simulink model "w31_v6"  (Simulink 7.9)
settings: Solver=FixedStepDiscrete  StartTime=0.0  StopTime=inf  FixedStep=0.01  RelTol=1e-3
undefined symbols (not defined in the file): DiscIntNeverNeededParam, magnitude
libraries: canmsglib x24, cansrvlib x22, simulink x12, iohwablib x5, legionoslib x3, ccpsrvlib x2, memsrvlib x1, tgttoollib x1, udssrvlib x1, wdgmlib x1
(part 5 of 5)

== stateflow chart CAN_Receive_10ms/Remote_Control_CAN/Remote_IO_situation1/Chart ==
  state MsgNotRecieve
    en:
    NoRxMsgComfirm=0;
    du:
    NoRxMsgCnt++;
  state MsgRecieve
    en:
    NoRxMsgCnt=0;
    NoRxMsgComfirm=0;
  state MsgNotRecieveComfirm
    en:
    NoRxMsgComfirm=1;
    du:
    NoRxMsgCnt++;
  note: NoRxMsgCnt在RxMsg==0的情况下（CAN信息没有在规定的周期内及时更新）
      | 一直往上加，直到RxMsg==1，NoRxMsgCnt清零。（程序接收到新的CAN信息）。NoRxMsgCnt只受到RxMsg控制。
  note: NoRxMsgComfirm受NoRxMsgCnt和NoRxMsgCntMax两个量控制
      | NoRxmsgComfirm==1没有接收到消息
  state NoRxMsgCntOverFlow
    en:
    NoRxMsgCnt=65000;
  (default) -> MsgNotRecieve : {NoRxMsgCnt=0;}
  MsgNotRecieve -> MsgRecieve [order 1] : [1==RxMsg]
  NoRxMsgCntOverFlow -> MsgRecieve : [1==RxMsg]
  MsgRecieve -> MsgNotRecieve : [0==RxMsg]
  MsgNotRecieveComfirm -> MsgRecieve [order 1] : [1==RxMsg]
  MsgNotRecieve -> MsgNotRecieveComfirm [order 2] : [NoRxMsgCnt>NoRxMsgCntMax]
  MsgNotRecieveComfirm -> NoRxMsgCntOverFlow [order 2] : [NoRxMsgCnt>=65000]
  data: NoRxMsgComfirm output boolean; RxMsg input boolean; NoRxMsgCnt output single; NoRxMsgCntMax input single

== stateflow chart CAN_Receive_10ms/Chassis_CAN/RL_Motor_NoMsg/Chart ==
  state MsgNotRecieve
    en:
    NoRxMsgComfirm=0;
    du:
    NoRxMsgCnt++;
  state MsgRecieve
    en:
    NoRxMsgCnt=0;
    NoRxMsgComfirm=0;
  state MsgNotRecieveComfirm
    en:
    NoRxMsgComfirm=1;
    du:
    NoRxMsgCnt++;
  note: NoRxMsgCnt在RxMsg==0的情况下（CAN信息没有在规定的周期内及时更新）
      | 一直往上加，直到RxMsg==1，NoRxMsgCnt清零。（程序接收到新的CAN信息）。NoRxMsgCnt只受到RxMsg控制。
  note: NoRxMsgComfirm受NoRxMsgCnt和NoRxMsgCntMax两个量控制
      | NoRxmsgComfirm==1没有接收到消息
  state NoRxMsgCntOverFlow
    en:
    NoRxMsgCnt=65000;
  (default) -> MsgNotRecieve : {NoRxMsgCnt=0;}
  MsgNotRecieve -> MsgRecieve [order 1] : [1==RxMsg]
  NoRxMsgCntOverFlow -> MsgRecieve : [1==RxMsg]
  MsgRecieve -> MsgNotRecieve : [0==RxMsg]
  MsgNotRecieveComfirm -> MsgRecieve [order 1] : [1==RxMsg]
  MsgNotRecieve -> MsgNotRecieveComfirm [order 2] : [NoRxMsgCnt>NoRxMsgCntMax]
  MsgNotRecieveComfirm -> NoRxMsgCntOverFlow [order 2] : [NoRxMsgCnt>=65000]
  data: NoRxMsgComfirm output boolean; RxMsg input boolean; NoRxMsgCnt output single; NoRxMsgCntMax input single

== stateflow chart CAN_Receive_10ms/Chassis_CAN/RR_Motor_NoMsg/Chart ==
  state MsgNotRecieve
    en:
    NoRxMsgComfirm=0;
    du:
    NoRxMsgCnt++;
  state MsgRecieve
    en:
    NoRxMsgCnt=0;
    NoRxMsgComfirm=0;
  state MsgNotRecieveComfirm
    en:
    NoRxMsgComfirm=1;
    du:
    NoRxMsgCnt++;
  note: NoRxMsgCnt在RxMsg==0的情况下（CAN信息没有在规定的周期内及时更新）
      | 一直往上加，直到RxMsg==1，NoRxMsgCnt清零。（程序接收到新的CAN信息）。NoRxMsgCnt只受到RxMsg控制。
  note: NoRxMsgComfirm受NoRxMsgCnt和NoRxMsgCntMax两个量控制
      | NoRxmsgComfirm==1没有接收到消息
  state NoRxMsgCntOverFlow
    en:
    NoRxMsgCnt=65000;
  (default) -> MsgNotRecieve : {NoRxMsgCnt=0;}
  MsgNotRecieve -> MsgRecieve [order 1] : [1==RxMsg]
  NoRxMsgCntOverFlow -> MsgRecieve : [1==RxMsg]
  MsgRecieve -> MsgNotRecieve : [0==RxMsg]
  MsgNotRecieveComfirm -> MsgRecieve [order 1] : [1==RxMsg]
  MsgNotRecieve -> MsgNotRecieveComfirm [order 2] : [NoRxMsgCnt>NoRxMsgCntMax]
  MsgNotRecieveComfirm -> NoRxMsgCntOverFlow [order 2] : [NoRxMsgCnt>=65000]
  data: NoRxMsgComfirm output boolean; RxMsg input boolean; NoRxMsgCnt output single; NoRxMsgCntMax input single

== matlab function Logic_And_Algorithm/Remote_mode_with_control_2/Power_calculation/Speed distribution strategy/speed gear slection ==
  data: u1 input double; y output double; u2 input double
function y = fcn(u1,u2)
%#codegen
%这个程序是用来做挡位控制的，目前希望是一档0-5，二档0-20，三档0-40.
if (u1==0)
    y = (5/30)*u2;

elseif(u1 == 1)
        y = (10/30)*u2;
        
else 
        y = (20/30)*u2;

end

y=u2;

end

== matlab function Logic_And_Algorithm/Remote_mode_with_control_0/Power_calculation/Speed distribution strategy/motion distribution1/Switch Case Action Subsystem/MATLAB Function ==
  data: steering_wheel_angle_dem input double; gain1 output double; gain2 output double; gain3 output double; gain4 output double
function [gain1,gain2,gain3,gain4] = fcn(steering_wheel_angle_dem)
%#codegen
%现进行逻辑说明，规定左转为正，右转为负，当前轮减后轮为正的时候，车辆左转，此时gain为逆时针原地转向；
%差值为负时，车辆右转，此时gain为顺时针原地转向

initial_gain=1;
gain1=initial_gain;
gain2=initial_gain;
gain3=initial_gain;
gain4=initial_gain;

if (steering_wheel_angle_dem>=0)
    gain1=-1;gain3=-1;
    gain2=1;gain4=1;
else
    gain1=1;gain3=1;
    gain2=-1;gain4=-1;
end

end

== stateflow chart CAN_Receive_10ms/iECU_CAN/shake_situation1/Chart ==
  state MsgNotRecieve
    en:
    NoRxMsgComfirm=0;
    du:
    NoRxMsgCnt++;
  state MsgRecieve
    en:
    NoRxMsgCnt=0;
    NoRxMsgComfirm=0;
  state MsgNotRecieveComfirm
    en:
    NoRxMsgComfirm=1;
    du:
    NoRxMsgCnt++;
  note: NoRxMsgCnt在RxMsg==0的情况下（CAN信息没有在规定的周期内及时更新）
      | 一直往上加，直到RxMsg==1，NoRxMsgCnt清零。（程序接收到新的CAN信息）。NoRxMsgCnt只受到RxMsg控制。
  note: NoRxMsgComfirm受NoRxMsgCnt和NoRxMsgCntMax两个量控制
      | NoRxmsgComfirm==1没有接收到消息
  state NoRxMsgCntOverFlow
    en:
    NoRxMsgCnt=65000;
  (default) -> MsgNotRecieve : {NoRxMsgCnt=0;}
  MsgNotRecieve -> MsgRecieve [order 1] : [1==RxMsg]
  NoRxMsgCntOverFlow -> MsgRecieve : [1==RxMsg]
  MsgRecieve -> MsgNotRecieve : [0==RxMsg]
  MsgNotRecieveComfirm -> MsgRecieve [order 1] : [1==RxMsg]
  MsgNotRecieve -> MsgNotRecieveComfirm [order 2] : [NoRxMsgCnt>NoRxMsgCntMax]
  MsgNotRecieveComfirm -> NoRxMsgCntOverFlow [order 2] : [NoRxMsgCnt>=65000]
  data: NoRxMsgComfirm output boolean; RxMsg input boolean; NoRxMsgCnt output single; NoRxMsgCntMax input single

== matlab function Logic_And_Algorithm/iECU_mode_with_control/Power_calculation/Speed distribution strategy/MATLAB Function ==
  data: u1 input double; y output double; u2 input double
function y = fcn(u1,u2)
%#codegen

if (u1 == 2 && u2 <= 20)
        y = u2;

elseif(u1 == 2 && u2 > 20)
        y = 20;        
        
elseif (u1==1 && u2 <= 10)
       y = u2;

elseif(u1 == 1 && u2 > 10)
        y = 10;    
        
elseif (u1==0 && u2 <= 5)
      y = u2;

else
       y = 5;            

end

== matlab function Logic_And_Algorithm/Remote_mode_with_control_0/Power_calculation/Speed distribution strategy/MATLAB Function ==
  data: delta_f input double; nan_code output double; delta_r input double; mode input double
function nan_code = fcn(delta_f,delta_r,mode)
%#codegen
%进行逻辑说明，如果判断在运算过程中会出现NAN的情况，则在此处将nan_code的值置为1，选择均分动力输出，
%否则nan_code=0，选择计算结果输出

initial_code=0;
nan_code=initial_code;

if (mode==0)&&(delta_f==delta_r)
    nan_code=1;
else if (mode==3)&&(delta_f==0)&&(delta_r==0)
        nan_code=1;
    else if (mode==2)&&(delta_r==0)
            nan_code=1;
        else if (mode==1)&&(delta_f==0)
                nan_code=1;
            else if (mode==4)
                    nan_code=0;
                
                end
            end
        end
    end
end

end

== stateflow chart CAN_Receive_10ms/BMS_CAN/shake_situation1/Chart ==
  state MsgNotRecieve
    en:
    NoRxMsgComfirm=0;
    du:
    NoRxMsgCnt++;
  state MsgRecieve
    en:
    NoRxMsgCnt=0;
    NoRxMsgComfirm=0;
  state MsgNotRecieveComfirm
    en:
    NoRxMsgComfirm=1;
    du:
    NoRxMsgCnt++;
  note: NoRxMsgCnt在RxMsg==0的情况下（CAN信息没有在规定的周期内及时更新）
      | 一直往上加，直到RxMsg==1，NoRxMsgCnt清零。（程序接收到新的CAN信息）。NoRxMsgCnt只受到RxMsg控制。
  note: NoRxMsgComfirm受NoRxMsgCnt和NoRxMsgCntMax两个量控制
      | NoRxmsgComfirm==1没有接收到消息
  state NoRxMsgCntOverFlow
    en:
    NoRxMsgCnt=65000;
  (default) -> MsgNotRecieve : {NoRxMsgCnt=0;}
  MsgNotRecieve -> MsgRecieve [order 1] : [1==RxMsg]
  NoRxMsgCntOverFlow -> MsgRecieve : [1==RxMsg]
  MsgRecieve -> MsgNotRecieve : [0==RxMsg]
  MsgNotRecieveComfirm -> MsgRecieve [order 1] : [1==RxMsg]
  MsgNotRecieve -> MsgNotRecieveComfirm [order 2] : [NoRxMsgCnt>NoRxMsgCntMax]
  MsgNotRecieveComfirm -> NoRxMsgCntOverFlow [order 2] : [NoRxMsgCnt>=65000]
  data: NoRxMsgComfirm output boolean; RxMsg input boolean; NoRxMsgCnt output single; NoRxMsgCntMax input single

== matlab function Logic_And_Algorithm/Remote_mode_with_control_0/Power_calculation/Speed distribution strategy/motion distribution1/front steering/MATLAB Function ==
  data: fl input double; motion_fl output double; fr input double; rl input double; rr input double; motion_dem input double; motion_fr output double; motion_rl output double; motion_rr output double
function [motion_fl,motion_fr,motion_rl,motion_rr] = fcn(fl,fr,rl,rr,motion_dem)
%#codegen
%逻辑说明，四轮的实际请求速度应该乘以4，所以此处有一个对应的语句，
%目前由于在前后轮转角输入都为0的情况下无法正常计算，输出会为NaN，因此在此进行判断，若有NaN的输出则均分动力

if isnan(fl)||isnan(fr)||isnan(rl)||isnan(rr)
    motion_fl=motion_dem;
    motion_fr=motion_dem;
    motion_rl=motion_dem;
    motion_rr=motion_dem;
else
    motion_fl=fl*4;
    motion_fr=fr*4;
    motion_rl=rl*4;
    motion_rr=rr*4;
end
end

== stateflow chart CAN_Receive_10ms/Chassis_CAN/DBSF_NoMsg/Chart ==
  state MsgNotRecieve
    en:
    NoRxMsgComfirm=0;
    du:
    NoRxMsgCnt++;
  state MsgRecieve
    en:
    NoRxMsgCnt=0;
    NoRxMsgComfirm=0;
  state MsgNotRecieveComfirm
    en:
    NoRxMsgComfirm=1;
    du:
    NoRxMsgCnt++;
  note: NoRxMsgCnt在RxMsg==0的情况下（CAN信息没有在规定的周期内及时更新）
      | 一直往上加，直到RxMsg==1，NoRxMsgCnt清零。（程序接收到新的CAN信息）。NoRxMsgCnt只受到RxMsg控制。
  note: NoRxMsgComfirm受NoRxMsgCnt和NoRxMsgCntMax两个量控制
      | NoRxmsgComfirm==1没有接收到消息
  state NoRxMsgCntOverFlow
    en:
    NoRxMsgCnt=65000;
  (default) -> MsgNotRecieve : {NoRxMsgCnt=0;}
  MsgNotRecieve -> MsgRecieve [order 1] : [1==RxMsg]
  NoRxMsgCntOverFlow -> MsgRecieve : [1==RxMsg]
  MsgRecieve -> MsgNotRecieve : [0==RxMsg]
  MsgNotRecieveComfirm -> MsgRecieve [order 1] : [1==RxMsg]
  MsgNotRecieve -> MsgNotRecieveComfirm [order 2] : [NoRxMsgCnt>NoRxMsgCntMax]
  MsgNotRecieveComfirm -> NoRxMsgCntOverFlow [order 2] : [NoRxMsgCnt>=65000]
  data: NoRxMsgComfirm output boolean; RxMsg input boolean; NoRxMsgCnt output single; NoRxMsgCntMax input single

== stateflow chart CAN_Receive_10ms/Chassis_CAN/EPSF_NoMsg/Chart ==
  state MsgNotRecieve
    en:
    NoRxMsgComfirm=0;
    du:
    NoRxMsgCnt++;
  state MsgRecieve
    en:
    NoRxMsgCnt=0;
    NoRxMsgComfirm=0;
  state MsgNotRecieveComfirm
    en:
    NoRxMsgComfirm=1;
    du:
    NoRxMsgCnt++;
  note: NoRxMsgCnt在RxMsg==0的情况下（CAN信息没有在规定的周期内及时更新）
      | 一直往上加，直到RxMsg==1，NoRxMsgCnt清零。（程序接收到新的CAN信息）。NoRxMsgCnt只受到RxMsg控制。
  note: NoRxMsgComfirm受NoRxMsgCnt和NoRxMsgCntMax两个量控制
      | NoRxmsgComfirm==1没有接收到消息
  state NoRxMsgCntOverFlow
    en:
    NoRxMsgCnt=65000;
  (default) -> MsgNotRecieve : {NoRxMsgCnt=0;}
  MsgNotRecieve -> MsgRecieve [order 1] : [1==RxMsg]
  NoRxMsgCntOverFlow -> MsgRecieve : [1==RxMsg]
  MsgRecieve -> MsgNotRecieve : [0==RxMsg]
  MsgNotRecieveComfirm -> MsgRecieve [order 1] : [1==RxMsg]
  MsgNotRecieve -> MsgNotRecieveComfirm [order 2] : [NoRxMsgCnt>NoRxMsgCntMax]
  MsgNotRecieveComfirm -> NoRxMsgCntOverFlow [order 2] : [NoRxMsgCnt>=65000]
  data: NoRxMsgComfirm output boolean; RxMsg input boolean; NoRxMsgCnt output single; NoRxMsgCntMax input single

== stateflow chart CAN_Receive_10ms/Chassis_CAN/EPSR_NoMsg/Chart ==
  state MsgNotRecieve
    en:
    NoRxMsgComfirm=0;
    du:
    NoRxMsgCnt++;
  state MsgRecieve
    en:
    NoRxMsgCnt=0;
    NoRxMsgComfirm=0;
  state MsgNotRecieveComfirm
    en:
    NoRxMsgComfirm=1;
    du:
    NoRxMsgCnt++;
  note: NoRxMsgCnt在RxMsg==0的情况下（CAN信息没有在规定的周期内及时更新）
      | 一直往上加，直到RxMsg==1，NoRxMsgCnt清零。（程序接收到新的CAN信息）。NoRxMsgCnt只受到RxMsg控制。
  note: NoRxMsgComfirm受NoRxMsgCnt和NoRxMsgCntMax两个量控制
      | NoRxmsgComfirm==1没有接收到消息
  state NoRxMsgCntOverFlow
    en:
    NoRxMsgCnt=65000;
  (default) -> MsgNotRecieve : {NoRxMsgCnt=0;}
  MsgNotRecieve -> MsgRecieve [order 1] : [1==RxMsg]
  NoRxMsgCntOverFlow -> MsgRecieve : [1==RxMsg]
  MsgRecieve -> MsgNotRecieve : [0==RxMsg]
  MsgNotRecieveComfirm -> MsgRecieve [order 1] : [1==RxMsg]
  MsgNotRecieve -> MsgNotRecieveComfirm [order 2] : [NoRxMsgCnt>NoRxMsgCntMax]
  MsgNotRecieveComfirm -> NoRxMsgCntOverFlow [order 2] : [NoRxMsgCnt>=65000]
  data: NoRxMsgComfirm output boolean; RxMsg input boolean; NoRxMsgCnt output single; NoRxMsgCntMax input single

== matlab function Logic_And_Algorithm/drive_mode_judegment/MATLAB Function ==
  data: remote_or_iECU input double; drive_mode output double; remote_speed_or_torque input double; iECU_control_flag input double
function drive_mode = fcn(remote_or_iECU,remote_speed_or_torque,iECU_control_flag)
%#codegen

%------------------------------------------------------------------------------------------
%进行判断的逻辑说明
%remote_or_iECU是遥控器按键B，用来判断是遥控控制还是iECU控制，按下为2，遥控控制，弹起为0，iECU控制
%上一步还需要结合iECU的指令来判断，当iECU_control_flag为0时，iECU没有发送请求，所以仍为遥控控制
%当iECU_control_flag为1且remote_or_iECU为0时，为iECU控制
%remote_speed_or_torque时遥控器按键A，按下为2，转矩直驱控制，弹起为0，转速控制
%drive_mode为1，iECU控制；为0，遥控转速控制；为2，遥控转矩控制
%横向数值为B键的remote_or_iECU,纵向数值为iECU_control_flag，drive_mode简化为mode
%         0               2
% 0       mode=A,遥控     mode=A,遥控
% 1       mode=1,iECU     mode=A,遥控
%----------------------------------------------------------------------------------------

initial_mode=uint8(2);
drive_mode=initial_mode;

if (remote_or_iECU==0)&&(iECU_control_flag==1)
    drive_mode=uint8(1);
else
    drive_mode=remote_speed_or_torque;
end

end

== matlab function Logic_And_Algorithm/Remote_mode_with_control_2/Power_calculation/Speed distribution strategy/truin_in_place_gain ==
  data: mode input double; gain1 output double; steer_angle input double; gain2 output double; gain3 output double; gain4 output double
function [gain1,gain2,gain3,gain4] = turn_in_place(mode,steer_angle)
%#codegen
%此模块为原地转向请求模块，在转角计算端输出转角信号为0，此处做顺时针或逆时针转向判断。
%当摇杆向左移动，输入的steer_angle为负值，以左侧为内侧进行转向；向右为正，以右侧为内侧进行转向
% 当mode==4时，进行此模块的判断，mode的数值来自于steer_calculation模块

%initializing
gain1=1;
gain2=1;
gain3=1;
gain4=1;

%表示遥控器关于原地转向的按键出现问题
% if mode~=4
%     error_code_turn_in_place=1;
% end

if (mode==4)&&(steer_angle<=0)
    gain1=-1;
    gain3=-1;
end

if (mode==4)&&(steer_angle>0)
    gain2=-1;
    gain4=-1;
end

end

== matlab function Logic_And_Algorithm/Remote_mode_with_control_2/Steering_calculation/Angle_Cal/Steer_Model_Judge/MATLAB Function ==
  data: steer_gear input double; mode output double; D_button input double
function mode = fcn(steer_gear,D_button)
%#codegen

%--------------------------------------------------------------------------
%进行逻辑说明：
% 横向为D_button,即D键的按键情况，0为未按下，2为按下
% 纵向为steer，即三档的转向模式开关，三档从左到右为0，1，2，具体数值需要测试确定
% *** 0                   2
% 0   mode=0,同向4WS      mode=3,反向4WS
% 1   mode=1,default,FS   
% 2   mode=2,RS           mode=4,原地转向
%--------------------------------------------------------------------------

initial_mode=1;
mode=initial_mode;

if (steer_gear==0)&&(D_button==0)
    mode=0;
end

if (steer_gear==0)&&(D_button==2)
    mode=3;
end

if (steer_gear==1)
    mode=1;
end

if (steer_gear==2)&&(D_button==0)
    mode=2;
end

if (steer_gear==2)&&(D_button==2)
    mode=4;
end

end

== matlab function Logic_And_Algorithm/Remote_mode_with_control_0/Power_calculation/Speed distribution strategy/motion distribution1/paralle steering/MATLAB Function ==
  data: fl input double; motion_fl output double; fr input double; rl input double; rr input double; motion_dem input double; motion_fr output double; motion_rl output double; motion_rr output double
function [motion_fl,motion_fr,motion_rl,motion_rr] = fcn(fl,fr,rl,rr,motion_dem)
%#codegen
%逻辑说明，四轮的实际请求速度应该乘以4，所以此处有一个对应的语句，
%目前由于在前后轮转角输入都为0的情况下无法正常计算，输出会为NaN，因此在此进行判断，若有NaN的输出则均分动力

if isnan(fl)||isnan(fr)||isnan(rl)||isnan(rr)
    motion_fl=motion_dem;
    motion_fr=motion_dem;
    motion_rl=motion_dem;
    motion_rr=motion_dem;
else
    motion_fl=fl*4;
    motion_fr=fr*4;
    motion_rl=rl*4;
    motion_rr=rr*4;
end
end

== matlab function Logic_And_Algorithm/Remote_mode_with_control_0/Power_calculation/Speed distribution strategy/motion distribution1/rear steering/MATLAB Function ==
  data: fl input double; motion_fl output double; fr input double; rl input double; rr input double; motion_dem input double; motion_fr output double; motion_rl output double; motion_rr output double
function [motion_fl,motion_fr,motion_rl,motion_rr] = fcn(fl,fr,rl,rr,motion_dem)
%#codegen
%逻辑说明，四轮的实际请求速度应该乘以4，所以此处有一个对应的语句，
%目前由于在前后轮转角输入都为0的情况下无法正常计算，输出会为NaN，因此在此进行判断，若有NaN的输出则均分动力

if isnan(fl)||isnan(fr)||isnan(rl)||isnan(rr)
    motion_fl=motion_dem;
    motion_fr=motion_dem;
    motion_rl=motion_dem;
    motion_rr=motion_dem;
else
    motion_fl=fl*4;
    motion_fr=fr*4;
    motion_rl=rl*4;
    motion_rr=rr*4;
end
end

== matlab function Logic_And_Algorithm/Remote_mode_with_control_0/Power_calculation/Speed distribution strategy/motion distribution1/reverse steering/MATLAB Function ==
  data: fl input double; motion_fl output double; fr input double; rl input double; rr input double; motion_dem input double; motion_fr output double; motion_rl output double; motion_rr output double
function [motion_fl,motion_fr,motion_rl,motion_rr] = fcn(fl,fr,rl,rr,motion_dem)
%#codegen
%逻辑说明，四轮的实际请求速度应该乘以4，所以此处有一个对应的语句，
%目前由于在前后轮转角输入都为0的情况下无法正常计算，输出会为NaN，因此在此进行判断，若有NaN的输出则均分动力

if isnan(fl)||isnan(fr)||isnan(rl)||isnan(rr)
    motion_fl=motion_dem;
    motion_fr=motion_dem;
    motion_rl=motion_dem;
    motion_rr=motion_dem;
else
    motion_fl=fl*4;
    motion_fr=fr*4;
    motion_rl=rl*4;
    motion_rr=rr*4;
end
end

== matlab function Logic_And_Algorithm/Remote_mode_with_control_0/Power_calculation/Speed distribution strategy/speed gear slection ==
  data: u1 input double; y output double; u2 input double
function y = fcn(u1,u2)
%#codegen
%这个程序是用来做挡位控制的，目前希望是一档0-5，二档0-20，三档0-40.
if (u1==0)
    y = (5/30)*u2;

elseif(u1 == 1)
        y = (10/30)*u2;
        
else 
        y = (20/30)*u2;

end

y=u2;

end

== matlab function Logic_And_Algorithm/Remote_mode_with_control_0/Steering_calculation/Angle_Cal/Steer_Model_Judge/MATLAB Function ==
  data: steer_gear input double; mode output double; D_button input double
function mode = fcn(steer_gear,D_button)
%#codegen

%--------------------------------------------------------------------------
%进行逻辑说明：
% 横向为D_button,即D键的按键情况，0为未按下，2为按下
% 纵向为steer，即三档的转向模式开关，三档从左到右为0，1，2，具体数值需要测试确定
% *** 0                   2
% 0   mode=0,同向4WS      mode=3,反向4WS
% 1   mode=1,default,FS   
% 2   mode=2,RS           mode=4,原地转向
%--------------------------------------------------------------------------

initial_mode=1;
mode=initial_mode;

if (steer_gear==0)&&(D_button==0)
    mode=0;
end

if (steer_gear==0)&&(D_button==2)
    mode=3;
end

if (steer_gear==1)
    mode=1;
end

if (steer_gear==2)&&(D_button==0)
    mode=2;
end

if (steer_gear==2)&&(D_button==2)
    mode=4;
end

end
